simulink model "model"  (R2013b)
settings: Solver=ode3  StartTime=9  StopTime=107  FixedStep=0.01  RelTol=1e-3
settings Model: Creator=Franta  LastModifiedBy=Franta

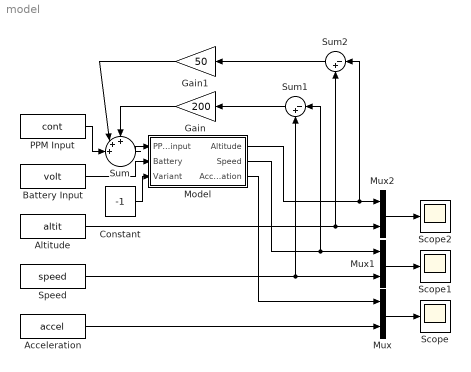
== system model ==
  Acceleration : FromWorkspace  VariableName=accel  SampleTime=0  OutputAfterFinalValue=Holding final value
  Altitude : FromWorkspace  VariableName=altit  SampleTime=0  OutputAfterFinalValue=Holding final value
  Battery Input : FromWorkspace  VariableName=volt  SampleTime=0  OutputAfterFinalValue=Holding final value
  Constant : Constant  Value=-1
  Gain : Gain  Gain=200
  Gain1 : Gain  Gain=50
  Model : Subsystem
  Mux : Mux  Inputs=2
  Mux1 : Mux  Inputs=2
  Mux2 : Mux  Inputs=2
  PPM Input : FromWorkspace  VariableName=cont  SampleTime=0  OutputAfterFinalValue=Holding final value
  Scope : Scope
      settings: YMin=0  YMax=47.5
  Scope1 : Scope
      settings: TimeRange=50
  Scope2 : Scope
      settings: SaveName=ScopeData2
  Speed : FromWorkspace  VariableName=speed  SampleTime=0  OutputAfterFinalValue=Holding final value
  Sum : Sum  Inputs=+++||
  Sum1 : Sum  Inputs=|-+
  Sum2 : Sum  Inputs=|-+
  wires:
  Mux/1 -> Scope/1
  Model/2(Speed) -> Mux1/1, Sum1/1
  Mux1/1 -> Scope1/1
  Model/3(Acceleration) -> Mux/1
  Speed/1 -> Mux1/2, Sum1/2
  Mux2/1 -> Scope2/1
  Model/1(Altitude) -> Sum2/1, Mux2/1
  Acceleration/1 -> Mux/2
  Sum/1 -> Model/1(PPM input)
  Gain/1 -> Sum/1
  Sum1/1 -> Gain/1
  PPM Input/1 -> Sum/3
  Sum2/1 -> Gain1/1
  Gain1/1 -> Sum/2
  Battery Input/1 -> Model/2(Battery)
  Altitude/1 -> Sum2/2, Mux2/2
  Constant/1 -> Model/3(Variant)

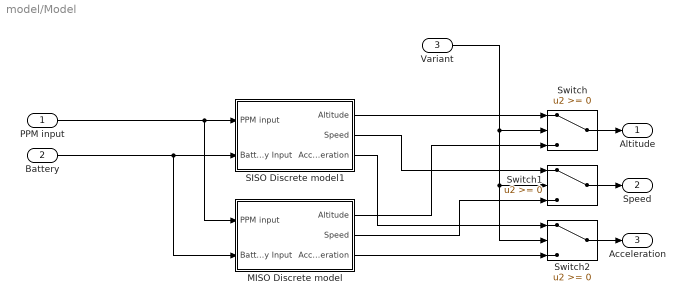
== system model/Model ==
  PPM input : Inport
  Battery : Inport  Port=2
  Variant : Inport  Port=3
  MISO Discrete model : Subsystem
  SISO Discrete model1 : Subsystem
  Switch : Switch
  Switch1 : Switch
  Switch2 : Switch
  Altitude : Outport
  Speed : Outport  Port=2
  Acceleration : Outport  Port=3
  wires:
  PPM input/1 -> MISO Discrete model/1(PPM input), SISO Discrete model1/1(PPM input)
  Battery/1 -> MISO Discrete model/2(Battery Input), SISO Discrete model1/2(Battery Input)
  Switch/1 -> Altitude/1
  Switch1/1 -> Speed/1
  Switch2/1 -> Acceleration/1
  SISO Discrete model1/1(Altitude) -> Switch/1
  MISO Discrete model/1(Altitude) -> Switch/3
  SISO Discrete model1/2(Speed) -> Switch1/1
  SISO Discrete model1/3(Acceleration) -> Switch2/1
  MISO Discrete model/2(Speed) -> Switch1/3
  MISO Discrete model/3(Acceleration) -> Switch2/3
  Variant/1 -> Switch2/2, Switch1/2, Switch/2

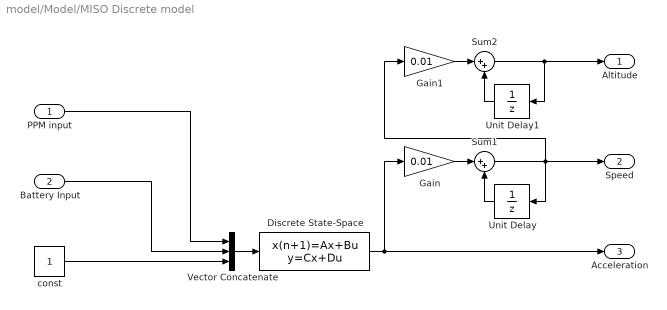
== system model/Model/MISO Discrete model ==
  PPM input : Inport
  Battery Input : Inport  Port=2
  Discrete State-Space : DiscreteStateSpace  A=[0.975860703201374 0.059286460158685;-0.042159733157818 0.939186054690820]  B=[6.314307851786213e-06 -4.754716441591897e-04 -0.035278240475003; 2.121430250334080e-05 0.007454859352531 -0.226118552362180]  C=[18.778733757834257 0.560758846210476]  D=[0 0 0]  SampleTime=0.01
  Gain : Gain  Gain=0.01
  Gain1 : Gain  Gain=0.01
  Sum1 : Sum  Inputs=|++
  Sum2 : Sum  Inputs=|++
  Unit Delay : UnitDelay  SampleTime=-1
  Unit Delay1 : UnitDelay  InitialCondition=1  SampleTime=-1
  Vector Concatenate : Concatenate  NumInputs=3
  const : Constant
  Altitude : Outport
  Speed : Outport  Port=2
  Acceleration : Outport  Port=3
  wires:
  Gain1/1 -> Sum2/1
  Gain/1 -> Sum1/1
  Unit Delay1/1 -> Sum2/2
  Sum2/1 -> Altitude/1, Unit Delay1/1
  Sum1/1 -> Speed/1, Gain1/1, Unit Delay/1
  Unit Delay/1 -> Sum1/2
  Discrete State-Space/1 -> Acceleration/1, Gain/1
  const/1 -> Vector Concatenate/3
  Battery Input/1 -> Vector Concatenate/2
  PPM input/1 -> Vector Concatenate/1
  Vector Concatenate/1 -> Discrete State-Space/1

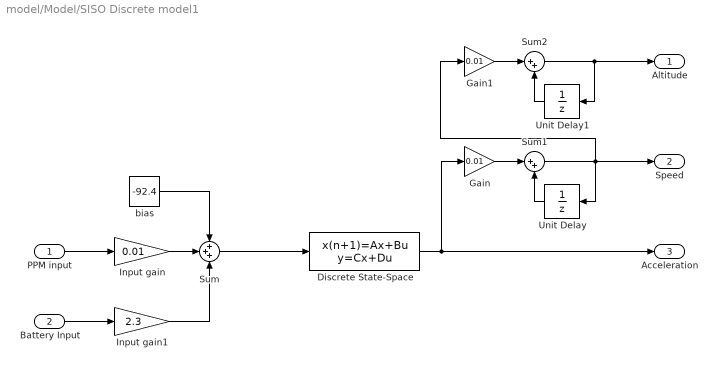
== system model/Model/SISO Discrete model1 ==
  PPM input : Inport
  Battery Input : Inport  Port=2
  Discrete State-Space : DiscreteStateSpace  A=[0.977737818067507 0.063938585278575;-0.039861855372271 0.932165964693411]  B=[0.001436277296681;0.003029732995050]  C=[10.627084380206110 0.333881682576147]  D=0  SampleTime=0.01
  Gain : Gain  Gain=0.01
  Gain1 : Gain  Gain=0.01
  Input gain : Gain  Gain=0.01
  Input gain1 : Gain  Gain=2.3
  Sum : Sum  Inputs=+++
  Sum1 : Sum  Inputs=|++
  Sum2 : Sum  Inputs=|++
  Unit Delay : UnitDelay  SampleTime=-1
  Unit Delay1 : UnitDelay  InitialCondition=1  SampleTime=-1
  bias : Constant  Value=-92.4
  Altitude : Outport
  Speed : Outport  Port=2
  Acceleration : Outport  Port=3
  wires:
  PPM input/1 -> Input gain/1
  Battery Input/1 -> Input gain1/1
  Input gain/1 -> Sum/2
  Input gain1/1 -> Sum/3
  bias/1 -> Sum/1
  Sum/1 -> Discrete State-Space/1
  Discrete State-Space/1 -> Gain/1, Acceleration/1
  Unit Delay/1 -> Sum1/2
  Sum1/1 -> Unit Delay/1, Gain1/1, Speed/1
  Sum2/1 -> Unit Delay1/1, Altitude/1
  Unit Delay1/1 -> Sum2/2
  Gain/1 -> Sum1/1
  Gain1/1 -> Sum2/1
